simulink model "posudesvodom"  (Simulink 6.6)
settings: Solver=ode45  StartTime=0.0  StopTime=16000  RelTol=1e-3
settings Model: Creator=Stjepan  LastModifiedBy=Stjepan

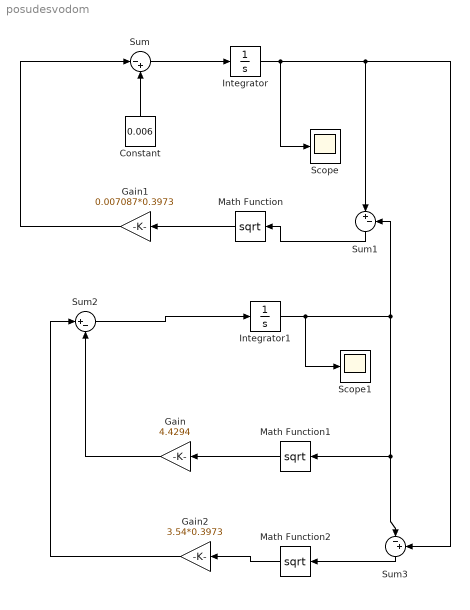
== system posudesvodom ==
  Constant : Constant  Orientation=up  Value=0.006
  Gain : Gain  Orientation=left  Gain=4.4294
  Gain1 : Gain  Orientation=left  Gain=0.007087*0.3973
  Gain2 : Gain  Orientation=left  Gain=3.54*0.3973
  Integrator : Integrator
  Integrator1 : Integrator
  Math Function : Math  Orientation=left  Operator=sqrt  SaturateOnIntegerOverflow=on
  Math Function1 : Math  Orientation=left  Operator=sqrt  SaturateOnIntegerOverflow=on
  Math Function2 : Math  Orientation=left  Operator=sqrt  SaturateOnIntegerOverflow=on
  Scope : Scope
      settings: TickLabels=on  TimeRange=16000  YMin=0  YMax=8  SampleInput=on  SampleTime=0.01
  Scope1 : Scope
      settings: TimeRange=16000  YMin=0  SampleInput=on  SampleTime=0.01
  Sum : Sum  Inputs=|-+
  Sum1 : Sum  Orientation=down  Inputs=|+-
  Sum2 : Sum  Inputs=|+-
  Sum3 : Sum  Orientation=down  Inputs=|-+
  wires:
  Constant/1 -> Sum/2
  Gain1/1 -> Sum/1
  Sum/1 -> Integrator/1
  Math Function/1 -> Gain1/1
  Integrator/1 -> Sum1/1, Sum3/2, Scope/1
  Sum1/1 -> Math Function/1
  Integrator1/1 -> Scope1/1, Sum1/2, Math Function1/1, Sum3/1
  Gain/1 -> Sum2/2
  Sum2/1 -> Integrator1/1
  Math Function1/1 -> Gain/1
  Gain2/1 -> Sum2/1
  Math Function2/1 -> Gain2/1
  Sum3/1 -> Math Function2/1
